simulink model "probnik_1"  (R2019a)
settings: Solver=FixedStepAuto  StartTime=0.0  StopTime=4  FixedStep=1e-5  RelTol=1e-3  EnableMultiTasking=on
values from neighbouring files (symbols this model uses):
  b1 = [3.31578564644 0.905199348927 -1.07588481903 -9.39754581451 6.51989841461 -7.39431810379 -7.98054647446 -7.51470994949 -2.46217346191 -2.60606265068 0.634998142719 -7.34759140015 ... (20 elements, 1x20)]    [b1.mat]
  b2 = [-8.908867836 -6.37810707092 -8.66125679016 -6.19361543655 -8.59416675568 -9.12425804138 -8.47231483459 -9.20506572723 -8.79118919373 -9.36305236816 -9.80707740784 -1.32926535606 ... (15 elements, 1x15)]    [b2.mat]
  b3 = 0.566753208637    [b3.mat]
  w1 = [-3.38608121872 -1.61282348633 -0.811974227428 -26.1486988068 -5.43596601486 -2.50496292114 -2.73406887054 -1.47529745102 -13.9745950699 -4.77835845947 -8.42057037354 -10.048833847 ... (100 elements, 5x20)]    [w1.mat]    (also in w1d.mat = [-28.5484638214 -28.3087368011 -16.2038860321 -18.8476390839)
  w2 = [-1.73702144623 -0.185042783618 -1.43662083149 5.53469181061 0.114013127983 -6.10858488083 1.57797574997 1.2862662077 -7.84612417221 -0.614148855209 -15.9998350143 -5.41085386276 ... (300 elements, 20x15)]    [w2.mat]    (also in w2d.mat = [-15.8134098053 -19.7163829803 -21.1157608032 -0.21424435079)
  w3 = [0.296215087175 2.04968070984 0.382735908031 1.65471422672 0.95603877306]    [w3.mat]    (also in w3d.mat = [-2.66624140739 1.28664553165 0.95645904541 -5.20410871506 2)
libraries: powerlib x33, simulink x14, powerlib_meascontrol x2, neural x2
settings Model: Creator=Андрей  LastModifiedBy=70810
settings DataIOCC: LimitDataPoints=on  SaveFormat=Array  ReturnWorkspaceOutputs=off
settings OptimizationCC: LifeSpan=inf
settings DebuggingCC: SolverPrmCheckMsg=warning  SFUnexpectedBacktrackingDiag=warning  SFNoUnconditionalDefaultTransitionDiag=warning  SFExecutionAtInitializationDiag=none  ArithmeticOperatorsInVariantConditions=warning
settings HardwareCC: ProdBitPerPointer=32  ProdBitPerSizeT=32  ProdBitPerPtrDiffT=32  ProdLargestAtomicFloat=None  ProdIntDivRoundTo=Undefined  ProdEndianess=Unspecified  ProdWordSize=32  ProdHWDeviceType=32-bit Generic
settings ModelReferenceCC: PropagateSignalLabelsOutOfModel=off
settings SFSimCC: SimUseLocalCustomCode=off
settings RTWCC: RTWUseLocalCustomCode=off
settings CodeAppCC: StateflowObjectComments=on
settings GRTTargetCC: TargetLangStandard=C89/C90 (ANSI)  GeneratePreprocessorConditionals=Disable all
settings ConfigComp: CovMetricSettings=dw  CovHtmlReporting=on  CovSaveCumulativeToWorkspaceVar=on  CovSaveSingleToWorkspaceVar=on  CovExternalEMLEnable=off  CovSFcnEnable=off
settings SimscapeCC: SimscapeNormalizeSystem=off

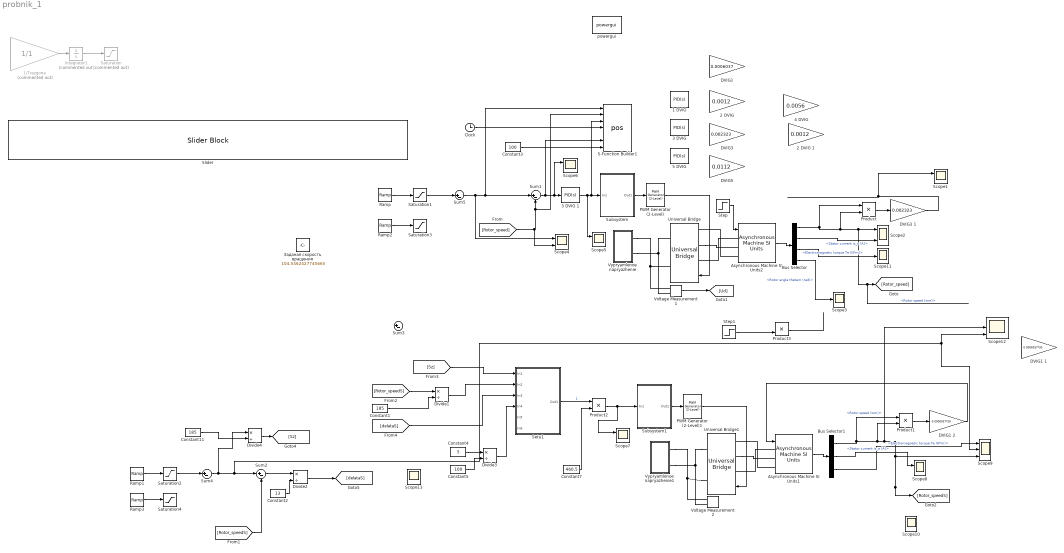
== system probnik_1 ==
  "1 DVIG " : simulink/Continuous/PID Controller  Controller=PID  Form=Parallel  TimeDomain=Continuous-time  SampleTime=-1  IntegratorMethod=Forward Euler  FilterMethod=Forward Euler  ControllerParametersSource=internal  P=1  I=60  D=0.004  UseFilter=on  N=100  TunerSelectOption=Transfer Function Based (PID Tuner App)  InitialConditionSource=internal  InitialConditionForIntegrator=0  InitialConditionForFilter=0  DifferentiatorICPrevScaledInput=0  ExternalReset=none  TrackingMode=off  Kt=1  LimitOutput=off  UpperSaturationLimit=inf  LowerSaturationLimit=-inf  LinearizeAsGain=on  AntiWindupMode=none  Kb=1  POutMin=[]  POutMax=[]  IOutMin=[]  IOutMax=[]  DOutMin=[]  DOutMax=[]  NOutMin=[]  NOutMax=[]  SumOutMin=[]  SumOutMax=[]  SaturationOutMin=[]  SaturationOutMax=[]  PParamMin=[]  PParamMax=[]  IParamMin=[]  IParamMax=[]  DParamMin=[]  DParamMax=[]  NParamMin=[]  NParamMax=[]  KbParamMin=[]  KbParamMax=[]  KtParamMin=[]  KtParamMax=[]  KbOutMin=[]  KbOutMax=[]  KtOutMin=[]  KtOutMax=[]  IntegratorOutMin=[]  IntegratorOutMax=[]  FilterOutMin=[]  FilterOutMax=[]  SumI1OutMin=[]  SumI1OutMax=[]  SumI2OutMin=[]  SumI2OutMax=[]  SumI3OutMin=[]  SumI3OutMax=[]  SumI4OutMin=[]  SumI4OutMax=[]  SumDOutMin=[]  SumDOutMax=[]  DifferentiatorOutMin=[]  DifferentiatorOutMax=[]  FilterDiffOutCoefMin=[]  FilterDiffOutCoefMax=[]  ReciprocalOutMin=[]  ReciprocalOutMax=[]  SumDenOutMin=[]  SumDenOutMax=[]  SumNumOutMin=[]  SumNumOutMax=[]  DivideOutMin=[]  DivideOutMax=[]  IntegratorContinuousStateAttributes=''  IntegratorStateMustResolveToSignalObject=off  IntegratorRTWStateStorageClass=Auto  FilterContinuousStateAttributes=''  FilterStateMustResolveToSignalObject=off  FilterRTWStateStorageClass=Auto  ParallelPVariant=InternalParameters  IdealPVariant=Disabled  IVariant=InternalParameters  DVariant=InternalParameters  IntegratorVariant=Continuous  SatVariant=Disabled  AWVariant=Passthrough  PCopyVariant=Disabled  TRVariant=Disabled  FdbkBlocksVariant=Forward  IdealPFdbkVariant=Disabled  SatFdbkVariant=Disabled  DerivativeFilterVariant=ContFilter  NVariant=InternalParameters  NCopyVariant=Disabled  FilterICVariant=InternalICsFilter  IntegratorICVariant=InternalICs  ExternalResetVariant=Disabled  TRSumVariant=Passthrough  SumFdbkVariant=Disabled  SumVariant=Sum_PID
  1/Trazgona : Gain  Commented=on  Gain=1/1
  "2 DVIG " : Gain  Gain=0.0012
  2 DVIG 1 : Gain  Gain=0.0012
  "3 DVIG " : simulink/Continuous/PID Controller  Controller=PID  Form=Parallel  TimeDomain=Continuous-time  SampleTime=-1  IntegratorMethod=Forward Euler  FilterMethod=Forward Euler  ControllerParametersSource=internal  P=1.8  I=35  D=0  UseFilter=on  N=100  TunerSelectOption=Transfer Function Based (PID Tuner App)  InitialConditionSource=internal  InitialConditionForIntegrator=0  InitialConditionForFilter=0  DifferentiatorICPrevScaledInput=0  ExternalReset=none  TrackingMode=off  Kt=1  LimitOutput=off  UpperSaturationLimit=inf  LowerSaturationLimit=-inf  LinearizeAsGain=on  AntiWindupMode=none  Kb=1  POutMin=[]  POutMax=[]  IOutMin=[]  IOutMax=[]  DOutMin=[]  DOutMax=[]  NOutMin=[]  NOutMax=[]  SumOutMin=[]  SumOutMax=[]  SaturationOutMin=[]  SaturationOutMax=[]  PParamMin=[]  PParamMax=[]  IParamMin=[]  IParamMax=[]  DParamMin=[]  DParamMax=[]  NParamMin=[]  NParamMax=[]  KbParamMin=[]  KbParamMax=[]  KtParamMin=[]  KtParamMax=[]  KbOutMin=[]  KbOutMax=[]  KtOutMin=[]  KtOutMax=[]  IntegratorOutMin=[]  IntegratorOutMax=[]  FilterOutMin=[]  FilterOutMax=[]  SumI1OutMin=[]  SumI1OutMax=[]  SumI2OutMin=[]  SumI2OutMax=[]  SumI3OutMin=[]  SumI3OutMax=[]  SumI4OutMin=[]  SumI4OutMax=[]  SumDOutMin=[]  SumDOutMax=[]  DifferentiatorOutMin=[]  DifferentiatorOutMax=[]  FilterDiffOutCoefMin=[]  FilterDiffOutCoefMax=[]  ReciprocalOutMin=[]  ReciprocalOutMax=[]  SumDenOutMin=[]  SumDenOutMax=[]  SumNumOutMin=[]  SumNumOutMax=[]  DivideOutMin=[]  DivideOutMax=[]  IntegratorContinuousStateAttributes=''  IntegratorStateMustResolveToSignalObject=off  IntegratorRTWStateStorageClass=Auto  FilterContinuousStateAttributes=''  FilterStateMustResolveToSignalObject=off  FilterRTWStateStorageClass=Auto  ParallelPVariant=InternalParameters  IdealPVariant=Disabled  IVariant=InternalParameters  DVariant=InternalParameters  IntegratorVariant=Continuous  SatVariant=Disabled  AWVariant=Passthrough  PCopyVariant=Disabled  TRVariant=Disabled  FdbkBlocksVariant=Forward  IdealPFdbkVariant=Disabled  SatFdbkVariant=Disabled  DerivativeFilterVariant=ContFilter  NVariant=InternalParameters  NCopyVariant=Disabled  FilterICVariant=InternalICsFilter  IntegratorICVariant=InternalICs  ExternalResetVariant=Disabled  TRSumVariant=Passthrough  SumFdbkVariant=Disabled  SumVariant=Sum_PID
  3 DVIG 1 : simulink/Continuous/PID Controller  Controller=PID  Form=Parallel  TimeDomain=Continuous-time  SampleTime=-1  IntegratorMethod=Forward Euler  FilterMethod=Forward Euler  ControllerParametersSource=internal  P=1.8  I=35  D=0  UseFilter=on  N=100  TunerSelectOption=Transfer Function Based (PID Tuner App)  InitialConditionSource=internal  InitialConditionForIntegrator=0  InitialConditionForFilter=0  DifferentiatorICPrevScaledInput=0  ExternalReset=none  TrackingMode=off  Kt=1  LimitOutput=off  UpperSaturationLimit=inf  LowerSaturationLimit=-inf  LinearizeAsGain=on  AntiWindupMode=none  Kb=1  POutMin=[]  POutMax=[]  IOutMin=[]  IOutMax=[]  DOutMin=[]  DOutMax=[]  NOutMin=[]  NOutMax=[]  SumOutMin=[]  SumOutMax=[]  SaturationOutMin=[]  SaturationOutMax=[]  PParamMin=[]  PParamMax=[]  IParamMin=[]  IParamMax=[]  DParamMin=[]  DParamMax=[]  NParamMin=[]  NParamMax=[]  KbParamMin=[]  KbParamMax=[]  KtParamMin=[]  KtParamMax=[]  KbOutMin=[]  KbOutMax=[]  KtOutMin=[]  KtOutMax=[]  IntegratorOutMin=[]  IntegratorOutMax=[]  FilterOutMin=[]  FilterOutMax=[]  SumI1OutMin=[]  SumI1OutMax=[]  SumI2OutMin=[]  SumI2OutMax=[]  SumI3OutMin=[]  SumI3OutMax=[]  SumI4OutMin=[]  SumI4OutMax=[]  SumDOutMin=[]  SumDOutMax=[]  DifferentiatorOutMin=[]  DifferentiatorOutMax=[]  FilterDiffOutCoefMin=[]  FilterDiffOutCoefMax=[]  ReciprocalOutMin=[]  ReciprocalOutMax=[]  SumDenOutMin=[]  SumDenOutMax=[]  SumNumOutMin=[]  SumNumOutMax=[]  DivideOutMin=[]  DivideOutMax=[]  IntegratorContinuousStateAttributes=''  IntegratorStateMustResolveToSignalObject=off  IntegratorRTWStateStorageClass=Auto  FilterContinuousStateAttributes=''  FilterStateMustResolveToSignalObject=off  FilterRTWStateStorageClass=Auto  ParallelPVariant=InternalParameters  IdealPVariant=Disabled  IVariant=InternalParameters  DVariant=InternalParameters  IntegratorVariant=Continuous  SatVariant=Disabled  AWVariant=Passthrough  PCopyVariant=Disabled  TRVariant=Disabled  FdbkBlocksVariant=Forward  IdealPFdbkVariant=Disabled  SatFdbkVariant=Disabled  DerivativeFilterVariant=ContFilter  NVariant=InternalParameters  NCopyVariant=Disabled  FilterICVariant=InternalICsFilter  IntegratorICVariant=InternalICs  ExternalResetVariant=Disabled  TRSumVariant=Passthrough  SumFdbkVariant=Disabled  SumVariant=Sum_PID
  "4 DVIG " : Gain  Gain=0.0056
  "5 DVIG " : simulink/Continuous/PID Controller  Controller=PID  Form=Parallel  TimeDomain=Continuous-time  SampleTime=-1  IntegratorMethod=Forward Euler  FilterMethod=Forward Euler  ControllerParametersSource=internal  P=2.3  I=33  D=0  UseFilter=on  N=100  TunerSelectOption=Transfer Function Based (PID Tuner App)  InitialConditionSource=internal  InitialConditionForIntegrator=0  InitialConditionForFilter=0  DifferentiatorICPrevScaledInput=0  ExternalReset=none  TrackingMode=off  Kt=1  LimitOutput=off  UpperSaturationLimit=inf  LowerSaturationLimit=-inf  LinearizeAsGain=on  AntiWindupMode=none  Kb=1  POutMin=[]  POutMax=[]  IOutMin=[]  IOutMax=[]  DOutMin=[]  DOutMax=[]  NOutMin=[]  NOutMax=[]  SumOutMin=[]  SumOutMax=[]  SaturationOutMin=[]  SaturationOutMax=[]  PParamMin=[]  PParamMax=[]  IParamMin=[]  IParamMax=[]  DParamMin=[]  DParamMax=[]  NParamMin=[]  NParamMax=[]  KbParamMin=[]  KbParamMax=[]  KtParamMin=[]  KtParamMax=[]  KbOutMin=[]  KbOutMax=[]  KtOutMin=[]  KtOutMax=[]  IntegratorOutMin=[]  IntegratorOutMax=[]  FilterOutMin=[]  FilterOutMax=[]  SumI1OutMin=[]  SumI1OutMax=[]  SumI2OutMin=[]  SumI2OutMax=[]  SumI3OutMin=[]  SumI3OutMax=[]  SumI4OutMin=[]  SumI4OutMax=[]  SumDOutMin=[]  SumDOutMax=[]  DifferentiatorOutMin=[]  DifferentiatorOutMax=[]  FilterDiffOutCoefMin=[]  FilterDiffOutCoefMax=[]  ReciprocalOutMin=[]  ReciprocalOutMax=[]  SumDenOutMin=[]  SumDenOutMax=[]  SumNumOutMin=[]  SumNumOutMax=[]  DivideOutMin=[]  DivideOutMax=[]  IntegratorContinuousStateAttributes=''  IntegratorStateMustResolveToSignalObject=off  IntegratorRTWStateStorageClass=Auto  FilterContinuousStateAttributes=''  FilterStateMustResolveToSignalObject=off  FilterRTWStateStorageClass=Auto  ParallelPVariant=InternalParameters  IdealPVariant=Disabled  IVariant=InternalParameters  DVariant=InternalParameters  IntegratorVariant=Continuous  SatVariant=Disabled  AWVariant=Passthrough  PCopyVariant=Disabled  TRVariant=Disabled  FdbkBlocksVariant=Forward  IdealPFdbkVariant=Disabled  SatFdbkVariant=Disabled  DerivativeFilterVariant=ContFilter  NVariant=InternalParameters  NCopyVariant=Disabled  FilterICVariant=InternalICsFilter  IntegratorICVariant=InternalICs  ExternalResetVariant=Disabled  TRSumVariant=Passthrough  SumFdbkVariant=Disabled  SumVariant=Sum_PID
  Asynchronous Machine SI Units1 : powerlib/Machines/Asynchronous Machine SI Units  RotorType=Squirrel-cage  PresetModel="06:  150 HP 460 V 60Hz 1785 RPM"  MechanicalLoad=Torque Tm  ShowDetailedParameters=on  ReferenceFrame=Rotor  Units=SI  MeasurementBus=off  NominalParameters=[1.119e+05 460 60]  Stator=[0.0302 0.000283]  Rotor=[0.01721 0.000283]  Cage1=[ 0.022 0.226/377]  Cage2=[ 0.022 0.226/377]  Lm=0.01095  Mechanical=[2 0.02154 2]  PolePairs=2  InitialConditions=[1 0 0 0 0 0 0 0]  SimulateSaturation=off  Saturation=[14.03593122, 27.81365428, 53.79336849, 72.68890987, 97.98006896, 148.6815601, 215.7428561, 302.9841135, 420.4778367 ; 230, 322, 414, 460, 506, 552, 598, 644, 690]  LoadFlowParameters=1492000  TsPowergui=0  TsBlock=-1  IterativeModel=Trapezoidal non iterative  IterativeDiscreteModel=Trapezoidal non iterative  Pmec=0
      settings: SourceProductName=Simscape Electrical
  Asynchronous Machine SI Units2 : powerlib/Machines/Asynchronous Machine SI Units  RotorType=Squirrel-cage  PresetModel="03:  20 HP  460 V 60Hz 1760 RPM"  MechanicalLoad=Torque Tm  ShowDetailedParameters=on  ReferenceFrame=Rotor  Units=SI  MeasurementBus=off  NominalParameters=[1.492e+04 460 60]  Stator=[0.2761 0.002191]  Rotor=[0.1645 0.002191]  Cage1=[ 0.022 0.226/377]  Cage2=[ 0.022 0.226/377]  Lm=0.07614  Mechanical=[0.1 0.01771 2]  PolePairs=2  InitialConditions=[1 0 0 0 0 0 0 0]  SimulateSaturation=off  Saturation=[14.03593122, 27.81365428, 53.79336849, 72.68890987, 97.98006896, 148.6815601, 215.7428561, 302.9841135, 420.4778367 ; 230, 322, 414, 460, 506, 552, 598, 644, 690]  LoadFlowParameters=1492000  TsPowergui=0  TsBlock=-1  IterativeModel=Trapezoidal non iterative  IterativeDiscreteModel=Trapezoidal non iterative  Pmec=0
      settings: SourceProductName=Simscape Electrical
  Bus Selector : BusSelector  OutputSignals=Mechanical.Rotor speed (wm),Stator measurements.Stator current is_a (A),Mechanical.Electromagnetic torque Te (N*m),Mechanical.Rotor angle thetam (rad)
  Bus Selector1 : BusSelector  OutputSignals=Mechanical.Rotor speed (wm),Stator measurements.Stator current is_a (A),Mechanical.Electromagnetic torque Te (N*m)
  Clock : Clock
  Constant1 : Constant  Value=185
  Constant11 : Constant  Value=185
  Constant2 : Constant  Value=13
  Constant3 : Constant  Value=100
  Constant4 : Constant  Value=5
  Constant5 : Constant  Value=100
  Constant7 : Constant  Value=460.5
  "DVIG1 " : Gain  Gain=0.0006037
  DVIG1 1 : Gain  Gain=0.0006037*30
  DVIG1 2 : Gain  Gain=0.0006037*30
  "DVIG3 " : Gain  Gain=0.002323
  DVIG3 1 : Gain  Gain=0.002323
  "DVIG5 " : Gain  Gain=0.0112
  Divide{1..4} (4 alike) : Product  Inputs=*/
  Integrator1 : Integrator  Commented=on
  PWM Generator (2-Level) : powerlib_meascontrol/Pulse & Signal Generators/PWM Generator (2-Level)  ModulatorType=Three-phase bridge (6 pulses)  ModulatorMode=Unsynchronized  Fc=1500  Pc=90  nF=27  MinMax="[ 0  1000 ]"  SamplingTechnique=Natural  ModulatingSignals=off  m=0.8  Freq=60  Phase=0  Ts=1e-5  ShowCarrierOutport=off
  PWM Generator (2-Level)1 : powerlib_meascontrol/Pulse & Signal Generators/PWM Generator (2-Level)  ModulatorType=Three-phase bridge (6 pulses)  ModulatorMode=Unsynchronized  Fc=1500  Pc=90  nF=27  MinMax="[ 0  1000 ]"  SamplingTechnique=Natural  ModulatingSignals=off  m=0.8  Freq=60  Phase=0  Ts=1e-5  ShowCarrierOutport=off
  Product{,1..3} (4 alike) : Product
  Ramp : simulink/Sources/Ramp  slope=183  start=0.1  InitialOutput=0
  Ramp1 : simulink/Sources/Ramp  slope=183  start=0.1  InitialOutput=0
  Ramp2 : simulink/Sources/Ramp  slope=183  start=1.5  InitialOutput=0
  Ramp3 : simulink/Sources/Ramp  slope=1830  start=1.6  InitialOutput=0
  S-Function Builder1 : S-Function  InitFcn=try, set_param(gcb,'FunctionName','pos'), end  FunctionName=pos  SFunctionModules=pos_wrapper Aray  SFunctionDeploymentMode=off  EnableBusSupport=off  mask(S-Function Builder){}
      mask help: Simulink:masks:SFunctionBuilder_MD
      mask init:
      | val = [[.9  0.75 0.75 1 1 .9 .9 1]',[1 1 0.75 0.75 .9 .9 1 .9]'];try , sys = get_param(gcb,'SfunBuilderFcnName');if isempty(sys), sys = get_param(gcb,'FunctionName'); end,catch, sys = get_param(gcb,'FunctionName'); end
      settings: CopyFcn=set_param(gcbh,'LinkStatus','none')  PreSaveFcn=try, set_param(gcb,'FunctionName','pos'), end  OpenFcn=sfunctionwizard(gcbh)
      mask Display: plot(val(:,1),val(:,2)),disp(sys), port_label('input',1,'u0'), port_label('input',2,'u1'), port_label('input',3,'u2'), port_label('input',4,'u3'), port_label('input',5,'u4'), port_label('input',6,'u5'), port_label('input',7,'u6'), port_label('output',1,'y0')
  Saturation : Saturate  Commented=on  UpperLimit=380  LowerLimit=0
  Saturation{1..4} (4 alike) : Saturate  UpperLimit=183  LowerLimit=0
  Scope{1..2,4..8,13} (8 alike) : Scope  NumInputPorts=2
  Scope10 : Scope
  Scope11 : Scope
  Scope12 : Scope  NumInputPorts=3
  Scope3 : Scope
  Scope9 : Scope  NumInputPorts=3
  Setu1 : Subsystem
  Slider : SliderBlock  ScaleMax=183
  Step : Step  Time=0.8  After=79  SampleTime=0
  Step1 : Step  Time=1.5  Before=1  After=0.1  SampleTime=0
  Subsystem : Subsystem
  Subsystem1 : Subsystem
  Sum{1..5} (5 alike) : Sum  Inputs=|+-
  Universal Bridge : powerlib/Power Electronics/Universal Bridge  Arms=3  SnubberResistance=1e5  SnubberCapacitance=inf  Device=IGBT / Diodes  Ron=1e-3  Lon=0  ForwardVoltages="[  0  0  ]"  ForwardVoltage=0  GTOparameters=[ 10e-6 , 20e-6 ]  IGBTparameters=[ 1e-6 , 2e-6 ]  Measurements=None  Measurements_2=None  converterType=Rectifier
      settings: SourceProductName=Simscape Electrical
  Universal Bridge1 : powerlib/Power Electronics/Universal Bridge  Arms=3  SnubberResistance=1e5  SnubberCapacitance=inf  Device=IGBT / Diodes  Ron=1e-3  Lon=0  ForwardVoltages="[  0  0  ]"  ForwardVoltage=0  GTOparameters=[ 10e-6 , 20e-6 ]  IGBTparameters=[ 1e-6 , 2e-6 ]  Measurements=None  Measurements_2=None  converterType=Rectifier
      settings: SourceProductName=Simscape Electrical
  Voltage Measurement1 : powerlib/Measurements/Voltage Measurement  PhasorSimulation=off  OutputType=Complex  PSBequivalent=0
      settings: SourceProductName=Simscape Electrical
  Voltage Measurement2 : powerlib/Measurements/Voltage Measurement  PhasorSimulation=off  OutputType=Complex  PSBequivalent=0
      settings: SourceProductName=Simscape Electrical
  Vypryamlenoe napryazhenie : Subsystem
  Vypryamlenoe napryazhenie1 : Subsystem
  powergui : powerlib/powergui  Priority=1  SimulationMode=Continuous  SampleTime=2e-5  frequency=60  Iterations=50  frequencyindice=0  Pbase=100e6  ErrMax=1e-4  UnitsV=kV  UnitsW=MW  buscounter=0  FunctionMessages=off  echomessages=off  EnableUseOfTLC=off  CurrentSourceSwitches=on  DisableSnubberDevices=off  DisableRonSwitches=off  DisableVfSwitches=off  DisplayEquations=off  AutomaticDiscreteSolvers=off  SolverType=Tustin  Interpol=off  ExternalGateDelay=off  methode=off  Ts=0  x0status=blocks  SPID=off  SwTol=0  HookPort=off  NonlinearTolerance=1e-4  nMaxIteration=100  ContinueOnMaxIteration=off  RestoreLinks=warning  ResistiveCurrentMeasurement=off  Frange=[0:2:500]  Ylog=off  Xlog=on  ShowGrid=off  save=off  variable=ZData  structure=0  ZoomFFT=off  StartTime=0.0  cycles=1  DisplayStyle=1  fundamental=60  FreqAxis=off  MaxFrequency=1000  frequencyindicesteady=1  RmsSteady=1  display=off
      settings: SourceProductName=Simscape Electrical
  "Заданая скорость вращения " : Constant  Value=104.5462427745665
  wires:
  Asynchronous Machine SI Units2/1 -> Bus Selector/1
  Product/1 -> DVIG3 1/1
  Bus Selector/3 -> Scope11/1  "<Electromagnetic torque Te (N*m)>"
  Bus Selector/1 -> Product/2, [Rotor_speed], Scope2/1, Product/1  "<Rotor speed (wm)>"
  DVIG3 1/1 -> Scope1/1
  Bus Selector/2 -> Scope2/2  "<Stator current is_a (A)>"
  PWM Generator (2-Level)/1 -> Universal Bridge/1
  Sum1/1 -> S-Function Builder1/6, 3 DVIG 1/1, Scope6/1
  [Rotor_speed] -> Scope4/2, S-Function Builder1/2, Sum1/2
  Voltage Measurement1/1 -> [Ud]
  Integrator1/1 -> Saturation/1
  1/Trazgona/1 -> Integrator1/1
  3 DVIG 1/1 -> Scope5/1, S-Function Builder1/3, Subsystem/1(In1)
  Subsystem/1(Out1) -> PWM Generator (2-Level)/1
  Ramp/1 -> Saturation1/1
  Bus Selector/4 -> Scope3/1  "<Rotor angle thetam (rad)>"
  Clock/1 -> S-Function Builder1/4
  PWM Generator (2-Level)1/1 -> Universal Bridge1/1
  Bus Selector1/3 -> Scope9/1  "<Electromagnetic torque Te (N*m)>"
  Subsystem1/1(Out1) -> PWM Generator (2-Level)1/1
  Bus Selector1/2 -> Scope8/1  "<Stator current is_a (A)>"
  Bus Selector1/1 -> Product1/1, Product1/2, Scope12/2, [Rotor_speedS], Scope9/3  "<Rotor speed (wm)>"
  Asynchronous Machine SI Units1/1 -> Bus Selector1/1
  Product1/1 -> DVIG1 2/1
  DVIG1 2/1 -> Asynchronous Machine SI Units1/1
  Setu1/1(Out1) -> Product2/1  "1"
  Constant7/1 -> Product2/2
  Constant11/1 -> Divide4/2
  Divide4/1 -> [Sz]
  Ramp1/1 -> Saturation2/1
  Sum2/1 -> Divide2/1
  [Rotor_speedS] -> Sum2/2
  [Rotor_speedS] -> Divide1/1
  Constant1/1 -> Divide1/2
  Divide1/1 -> Setu1/2(In2)
  [Sz] -> Setu1/1(In1)
  Constant2/1 -> Divide2/2
  Divide2/1 -> [delataS]
  [delataS] -> Setu1/3(In3)
  Product2/1 -> Scope7/1, Subsystem1/1(In1)
  Saturation2/1 -> Sum4/1
  Sum4/1 -> Divide4/1, Scope9/2, Scope12/3, Sum2/1
  Saturation1/1 -> Sum5/1
  Sum5/1 -> Scope4/1, S-Function Builder1/1, Sum1/1
  Constant3/1 -> S-Function Builder1/7
  Constant4/1 -> Divide3/1
  Constant5/1 -> Divide3/2
  Divide3/1 -> Setu1/4(In4)
  Ramp2/1 -> Saturation3/1
  Ramp3/1 -> Saturation4/1
  Step/1 -> Asynchronous Machine SI Units2/1
  Step1/1 -> Product3/2
  Product3/1 -> ?
  connections:
  Asynchronous Machine SI Units2/LConn1 -- Universal Bridge/LConn1
  Asynchronous Machine SI Units2/LConn3 -- Universal Bridge/LConn3
  Universal Bridge/LConn2 -- Asynchronous Machine SI Units2/LConn2
  Vypryamlenoe napryazhenie/RConn2 -- Voltage Measurement1/LConn2 -- Universal Bridge/RConn2
  Voltage Measurement1/LConn1 -- Vypryamlenoe napryazhenie/RConn1 -- Universal Bridge/RConn1
  Universal Bridge1/RConn1 -- Voltage Measurement2/LConn1 -- Vypryamlenoe napryazhenie1/RConn1
  Universal Bridge1/RConn2 -- Vypryamlenoe napryazhenie1/RConn2 -- Voltage Measurement2/LConn2
  Asynchronous Machine SI Units1/LConn1 -- Universal Bridge1/LConn1
  Universal Bridge1/LConn2 -- Asynchronous Machine SI Units1/LConn2
  Asynchronous Machine SI Units1/LConn3 -- Universal Bridge1/LConn3

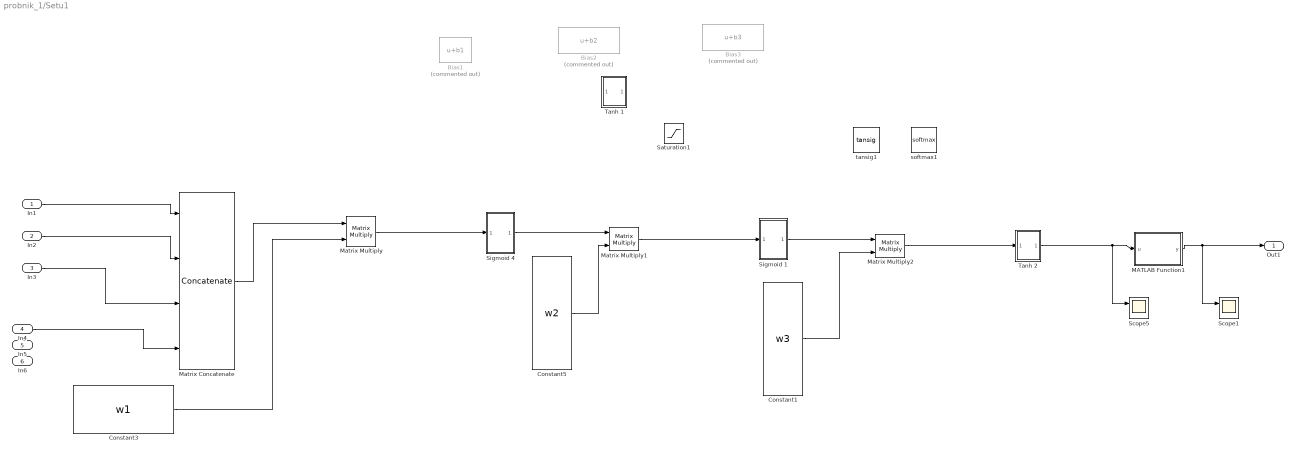
== system probnik_1/Setu1 ==
  In1 : Inport
  In2 : Inport  Port=2
  In3 : Inport  Port=3
  In4 : Inport  Port=4
  In5 : Inport  Port=5
  In6 : Inport  Port=6
  Bias1 : Bias  Commented=on  Bias=b1
  Bias2 : Bias  Commented=on  Bias=b2
  Bias3 : Bias  Commented=on  Bias=b3
  Constant1 : Constant  Value=w3  VectorParams1D=off
  Constant3 : Constant  Value=w1  VectorParams1D=off
  Constant5 : Constant  Value=w2  VectorParams1D=off
  MATLAB Function1 : MATLAB Function  TreatAsAtomicUnit=on
  Matrix Concatenate : Concatenate  NumInputs=4  Mode=Multidimensional array  ConcatenateDimension=2
  Matrix Multiply : Product  Multiplication=Matrix(*)
  Matrix Multiply1 : Product  Multiplication=Matrix(*)
  Matrix Multiply2 : Product  Multiplication=Matrix(*)
  Saturation1 : Saturate  UpperLimit=inf  LowerLimit=0
  Scope1 : Scope  NumInputPorts=2
  Scope5 : Scope  NumInputPorts=2
  Sigmoid 1 : Subsystem
  Sigmoid 4 : Subsystem
  Tanh 1 : Subsystem
  Tanh 2 : Subsystem
  softmax1 : neural/Transfer Functions/softmax
      settings: SourceProductName=MATLAB Runtime - Deep Learning Toolbox  SourceProductBaseCode=Missing
  tansig1 : neural/Transfer Functions/tansig
      settings: SourceProductName=MATLAB Runtime - Deep Learning Toolbox  SourceProductBaseCode=Missing
  Out1 : Outport
  wires:
  Sigmoid 4/1(Out1) -> Matrix Multiply1/1
  Sigmoid 1/1(Out1) -> Matrix Multiply2/1
  Constant1/1 -> Matrix Multiply2/2
  Constant3/1 -> Matrix Multiply/2
  Constant5/1 -> Matrix Multiply1/2
  In1/1 -> Matrix Concatenate/1
  Matrix Concatenate/1 -> Matrix Multiply/1
  In2/1 -> Matrix Concatenate/2
  In3/1 -> Matrix Concatenate/3
  In4/1 -> Matrix Concatenate/4
  Matrix Multiply/1 -> Sigmoid 4/1(In1)
  Matrix Multiply1/1 -> Sigmoid 1/1(In1)
  Matrix Multiply2/1 -> Tanh 2/1(In1)
  Tanh 2/1(Out1) -> MATLAB Function1/1(u), Scope5/1
  MATLAB Function1/1(y) -> Scope1/1, Out1/1

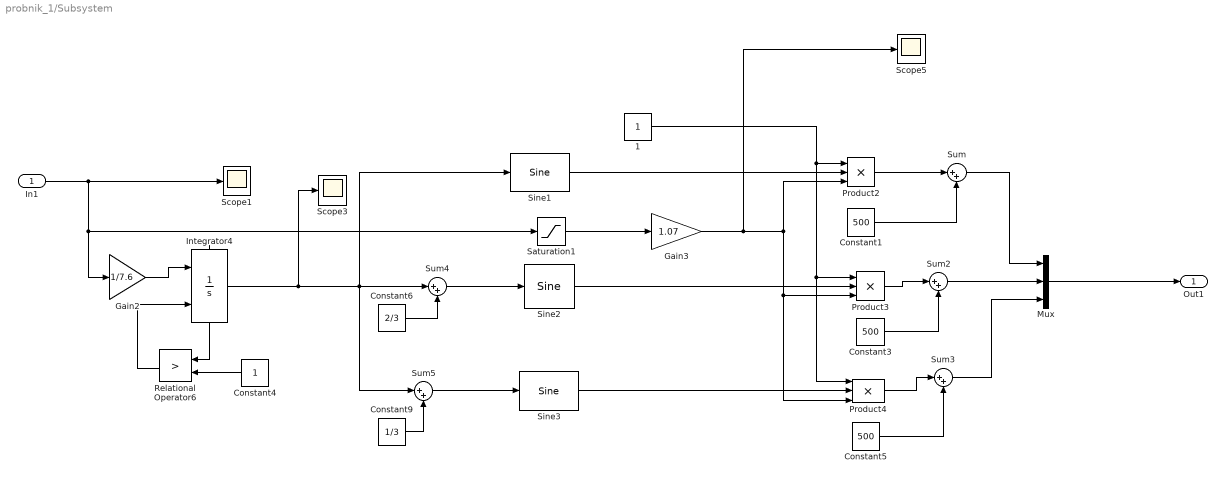
== system probnik_1/Subsystem ==
  In1 : Inport
  " 1" : Constant
  Constant1 : Constant  Value=500
  Constant3 : Constant  Value=500
  Constant4 : Constant
  Constant5 : Constant  Value=500
  Constant6 : Constant  Value=2/3
  Constant9 : Constant  Value=1/3
  Gain2 : Gain  Gain=1/7.6
  Gain3 : Gain  Gain=1.07
  Integrator4 : Integrator  ExternalReset=rising  ShowStatePort=on
  Mux : Mux  Inputs=3
  Product2 : Product  Inputs=3
  Product3 : Product  Inputs=3
  Product4 : Product  Inputs=3
  Relational Operator6 : RelationalOperator  Operator=>  RndMeth=Nearest  InputSameDT=on
  Saturation1 : Saturate  UpperLimit=650  LowerLimit=-650
  Scope1 : Scope
  Scope3 : Scope
  Scope5 : Scope
  Sine1 : simulink/Lookup Tables/Sine  Formula=sin(2*pi*u)  NumDataPoints=(2^5)+1  OutputWordLength=16  InternalRulePriority=Speed
      settings: SourceProductName=Simulink
  Sine2 : simulink/Lookup Tables/Sine  Formula=sin(2*pi*u)  NumDataPoints=(2^5)+1  OutputWordLength=16  InternalRulePriority=Speed
      settings: SourceProductName=Simulink
  Sine3 : simulink/Lookup Tables/Sine  Formula=sin(2*pi*u)  NumDataPoints=(2^5)+1  OutputWordLength=16  InternalRulePriority=Speed
      settings: SourceProductName=Simulink
  Sum{,2..5} (5 alike) : Sum  Inputs=|++
  Out1 : Outport
  wires:
  In1/1 -> Saturation1/1, Gain2/1, Scope1/1
  Integrator4/State -> Relational Operator6/1
  Gain3/1 -> Scope5/1, Product2/3, Product4/3, Product3/3
  Relational Operator6/1 -> Integrator4/2
  Product3/1 -> Sum2/1
  Constant5/1 -> Sum3/2
  Sine1/1 -> Product2/2
  Sine2/1 -> Product3/2
  Product4/1 -> Sum3/1
  Constant6/1 -> Sum4/2
  Constant1/1 -> Sum/2
  Constant9/1 -> Sum5/2
  Sum4/1 -> Sine2/1
  Sum5/1 -> Sine3/1
  Gain2/1 -> Integrator4/1
  Sum3/1 -> Mux/3
  Sum/1 -> Mux/1
  Constant4/1 -> Relational Operator6/2
  Constant3/1 -> Sum2/2
  Sine3/1 -> Product4/2
  Integrator4/1 -> Scope3/1, Sine1/1, Sum5/1, Sum4/1
  Saturation1/1 -> Gain3/1
  Sum2/1 -> Mux/2
  Product2/1 -> Sum/1
  " 1"/1 -> Product4/1, Product3/1, Product2/1
  Mux/1 -> Out1/1

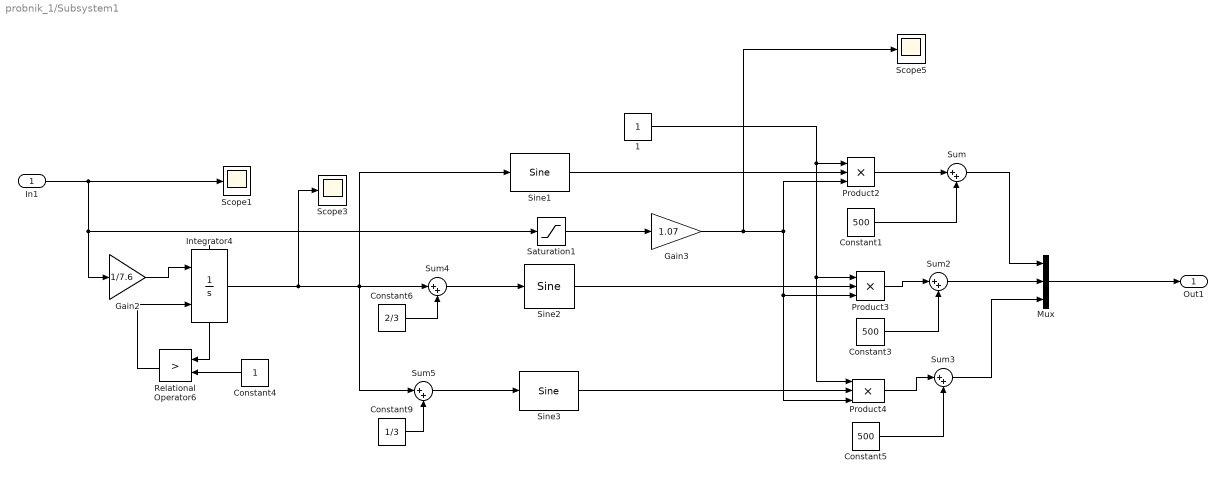
== system probnik_1/Subsystem1 ==
  In1 : Inport
  " 1" : Constant
  Constant1 : Constant  Value=500
  Constant3 : Constant  Value=500
  Constant4 : Constant
  Constant5 : Constant  Value=500
  Constant6 : Constant  Value=2/3
  Constant9 : Constant  Value=1/3
  Gain2 : Gain  Gain=1/7.6
  Gain3 : Gain  Gain=1.07
  Integrator4 : Integrator  ExternalReset=rising  ShowStatePort=on
  Mux : Mux  Inputs=3
  Product2 : Product  Inputs=3
  Product3 : Product  Inputs=3
  Product4 : Product  Inputs=3
  Relational Operator6 : RelationalOperator  Operator=>  RndMeth=Nearest  InputSameDT=on
  Saturation1 : Saturate  UpperLimit=650  LowerLimit=-650
  Scope1 : Scope
  Scope3 : Scope
  Scope5 : Scope
  Sine1 : simulink/Lookup Tables/Sine  Formula=sin(2*pi*u)  NumDataPoints=(2^5)+1  OutputWordLength=16  InternalRulePriority=Speed
      settings: SourceProductName=Simulink
  Sine2 : simulink/Lookup Tables/Sine  Formula=sin(2*pi*u)  NumDataPoints=(2^5)+1  OutputWordLength=16  InternalRulePriority=Speed
      settings: SourceProductName=Simulink
  Sine3 : simulink/Lookup Tables/Sine  Formula=sin(2*pi*u)  NumDataPoints=(2^5)+1  OutputWordLength=16  InternalRulePriority=Speed
      settings: SourceProductName=Simulink
  Sum{,2..5} (5 alike) : Sum  Inputs=|++
  Out1 : Outport
  wires:
  In1/1 -> Saturation1/1, Gain2/1, Scope1/1
  Integrator4/State -> Relational Operator6/1
  Gain3/1 -> Scope5/1, Product2/3, Product4/3, Product3/3
  Relational Operator6/1 -> Integrator4/2
  Product3/1 -> Sum2/1
  Constant5/1 -> Sum3/2
  Sine1/1 -> Product2/2
  Sine2/1 -> Product3/2
  Product4/1 -> Sum3/1
  Constant6/1 -> Sum4/2
  Constant1/1 -> Sum/2
  Constant9/1 -> Sum5/2
  Sum4/1 -> Sine2/1
  Sum5/1 -> Sine3/1
  Gain2/1 -> Integrator4/1
  Sum3/1 -> Mux/3
  Sum/1 -> Mux/1
  Constant4/1 -> Relational Operator6/2
  Constant3/1 -> Sum2/2
  Sine3/1 -> Product4/2
  Integrator4/1 -> Scope3/1, Sine1/1, Sum5/1, Sum4/1
  Saturation1/1 -> Gain3/1
  Sum2/1 -> Mux/2
  Product2/1 -> Sum/1
  " 1"/1 -> Product4/1, Product3/1, Product2/1
  Mux/1 -> Out1/1

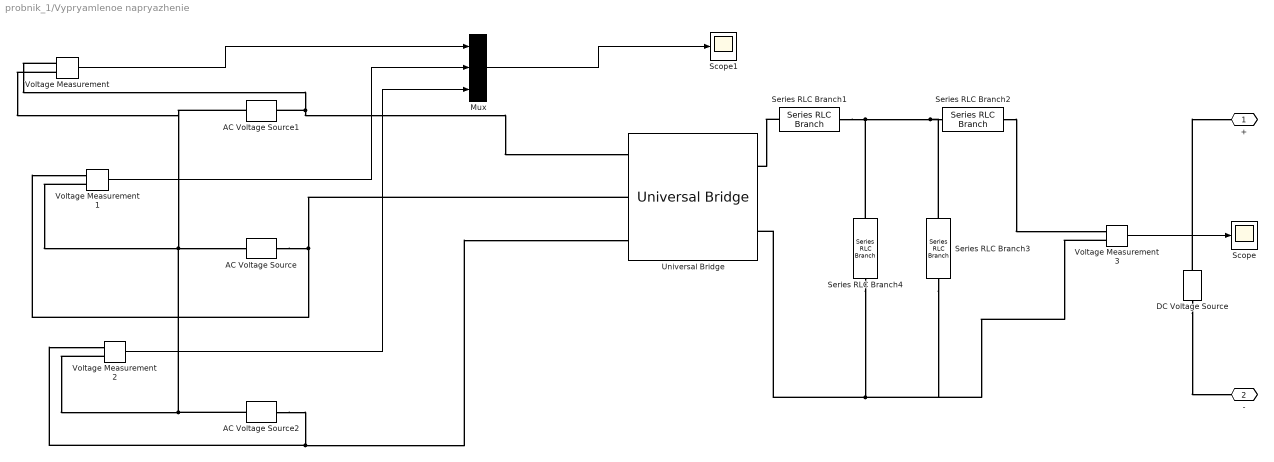
== system probnik_1/Vypryamlenoe napryazhenie ==
  AC Voltage Source : powerlib/Electrical Sources/AC Voltage Source  Amplitude=460  Phase=120  Frequency=120  SampleTime=0  Measurements=None  BusType=swing  Pref=10e3  Qref=0  Qmin=-inf  Qmax=+inf
      settings: SourceProductName=Simscape Electrical
  AC Voltage Source1 : powerlib/Electrical Sources/AC Voltage Source  Amplitude=460  Phase=0  Frequency=120  SampleTime=0  Measurements=None  BusType=swing  Pref=10e3  Qref=0  Qmin=-inf  Qmax=+inf
      settings: SourceProductName=Simscape Electrical
  AC Voltage Source2 : powerlib/Electrical Sources/AC Voltage Source  Amplitude=460  Phase=240  Frequency=120  SampleTime=0  Measurements=None  BusType=swing  Pref=10e3  Qref=0  Qmin=-inf  Qmax=+inf
      settings: SourceProductName=Simscape Electrical
  DC Voltage Source : powerlib/Electrical Sources/DC Voltage Source  Amplitude=900  Measurements=None
      settings: SourceProductName=Simscape Electrical
  Mux : Mux  Inputs=3
  Scope : Scope
  Scope1 : Scope
  Series RLC Branch1 : powerlib/Elements/Series RLC Branch  LConnTagsString=__new0  RConnTagsString=__new0  BranchType=R  Resistance=0.01  Inductance=1e-3  SetiL0=off  InitialCurrent=0  Capacitance=1e-3  Setx0=off  InitialVoltage=0  Measurements=None
      settings: SourceProductName=Simscape Electrical
  Series RLC Branch2 : powerlib/Elements/Series RLC Branch  LConnTagsString=__new0  RConnTagsString=__new0  BranchType=R  Resistance=0.01  Inductance=1e-3  SetiL0=off  InitialCurrent=0  Capacitance=1e-3  Setx0=off  InitialVoltage=0  Measurements=None
      settings: SourceProductName=Simscape Electrical
  Series RLC Branch3 : powerlib/Elements/Series RLC Branch  LConnTagsString=__new0  RConnTagsString=__new0  BranchType=C  Resistance=100  Inductance=1e-3  SetiL0=off  InitialCurrent=0  Capacitance=3e-3  Setx0=off  InitialVoltage=0  Measurements=None
      settings: SourceProductName=Simscape Electrical
  Series RLC Branch4 : powerlib/Elements/Series RLC Branch  LConnTagsString=__new0  RConnTagsString=__new0  BranchType=R  Resistance=1  Inductance=1e-3  SetiL0=off  InitialCurrent=0  Capacitance=1e-3  Setx0=off  InitialVoltage=0  Measurements=None
      settings: SourceProductName=Simscape Electrical
  Universal Bridge : powerlib/Power Electronics/Universal Bridge  Arms=3  SnubberResistance=1e5  SnubberCapacitance=inf  Device=Diodes  Ron=1e-3  Lon=0  ForwardVoltages="[  0  0  ]"  ForwardVoltage=0  GTOparameters=[ 10e-6 , 20e-6 ]  IGBTparameters=[ 1e-6 , 2e-6 ]  Measurements=None  Measurements_2=None  converterType=Rectifier
      settings: SourceProductName=Simscape Electrical
  Voltage Measurement{,1..3} (4 alike) : powerlib/Measurements/Voltage Measurement  PhasorSimulation=off  OutputType=Complex  PSBequivalent=0
      settings: SourceProductName=Simscape Electrical
  + : PMIOPort  Side=Right
  - : PMIOPort  Port=2  Side=Right
  wires:
  Voltage Measurement/1 -> Mux/1
  Voltage Measurement2/1 -> Mux/3
  Mux/1 -> Scope1/1
  Voltage Measurement1/1 -> Mux/2
  Voltage Measurement3/1 -> Scope/1
  connections:
  AC Voltage Source2/LConn1 -- Voltage Measurement/LConn2 -- AC Voltage Source1/LConn1 -- AC Voltage Source/LConn1 -- Voltage Measurement1/LConn2 -- Voltage Measurement2/LConn2
  AC Voltage Source2/RConn1 -- Universal Bridge/LConn3 -- Voltage Measurement2/LConn1
  Voltage Measurement3/LConn2 -- Series RLC Branch3/LConn1 -- Series RLC Branch4/LConn1 -- Universal Bridge/RConn2
  AC Voltage Source/RConn1 -- Voltage Measurement1/LConn1 -- Universal Bridge/LConn2
  Series RLC Branch1/LConn1 -- Series RLC Branch4/RConn1 -- Series RLC Branch3/RConn1 -- Series RLC Branch2/RConn1
  Series RLC Branch2/LConn1 -- Voltage Measurement3/LConn1
  Voltage Measurement/LConn1 -- Universal Bridge/LConn1 -- AC Voltage Source1/RConn1
  Series RLC Branch1/RConn1 -- Universal Bridge/RConn1
  DC Voltage Source/RConn1 -- +/RConn1
  DC Voltage Source/LConn1 -- -/RConn1

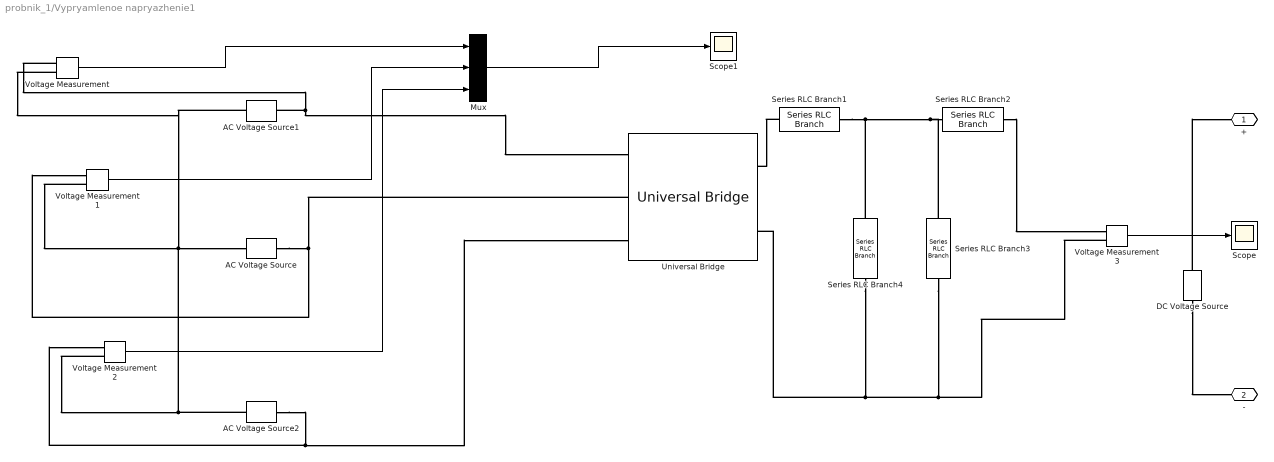
== system probnik_1/Vypryamlenoe napryazhenie1 ==
  AC Voltage Source : powerlib/Electrical Sources/AC Voltage Source  Amplitude=460  Phase=120  Frequency=120  SampleTime=0  Measurements=None  BusType=swing  Pref=10e3  Qref=0  Qmin=-inf  Qmax=+inf
      settings: SourceProductName=Simscape Electrical
  AC Voltage Source1 : powerlib/Electrical Sources/AC Voltage Source  Amplitude=460  Phase=0  Frequency=120  SampleTime=0  Measurements=None  BusType=swing  Pref=10e3  Qref=0  Qmin=-inf  Qmax=+inf
      settings: SourceProductName=Simscape Electrical
  AC Voltage Source2 : powerlib/Electrical Sources/AC Voltage Source  Amplitude=460  Phase=240  Frequency=120  SampleTime=0  Measurements=None  BusType=swing  Pref=10e3  Qref=0  Qmin=-inf  Qmax=+inf
      settings: SourceProductName=Simscape Electrical
  DC Voltage Source : powerlib/Electrical Sources/DC Voltage Source  Amplitude=900  Measurements=None
      settings: SourceProductName=Simscape Electrical
  Mux : Mux  Inputs=3
  Scope : Scope
  Scope1 : Scope
  Series RLC Branch1 : powerlib/Elements/Series RLC Branch  LConnTagsString=__new0  RConnTagsString=__new0  BranchType=R  Resistance=0.01  Inductance=1e-3  SetiL0=off  InitialCurrent=0  Capacitance=1e-3  Setx0=off  InitialVoltage=0  Measurements=None
      settings: SourceProductName=Simscape Electrical
  Series RLC Branch2 : powerlib/Elements/Series RLC Branch  LConnTagsString=__new0  RConnTagsString=__new0  BranchType=R  Resistance=0.01  Inductance=1e-3  SetiL0=off  InitialCurrent=0  Capacitance=1e-3  Setx0=off  InitialVoltage=0  Measurements=None
      settings: SourceProductName=Simscape Electrical
  Series RLC Branch3 : powerlib/Elements/Series RLC Branch  LConnTagsString=__new0  RConnTagsString=__new0  BranchType=C  Resistance=100  Inductance=1e-3  SetiL0=off  InitialCurrent=0  Capacitance=3e-3  Setx0=off  InitialVoltage=0  Measurements=None
      settings: SourceProductName=Simscape Electrical
  Series RLC Branch4 : powerlib/Elements/Series RLC Branch  LConnTagsString=__new0  RConnTagsString=__new0  BranchType=R  Resistance=1  Inductance=1e-3  SetiL0=off  InitialCurrent=0  Capacitance=1e-3  Setx0=off  InitialVoltage=0  Measurements=None
      settings: SourceProductName=Simscape Electrical
  Universal Bridge : powerlib/Power Electronics/Universal Bridge  Arms=3  SnubberResistance=1e5  SnubberCapacitance=inf  Device=Diodes  Ron=1e-3  Lon=0  ForwardVoltages="[  0  0  ]"  ForwardVoltage=0  GTOparameters=[ 10e-6 , 20e-6 ]  IGBTparameters=[ 1e-6 , 2e-6 ]  Measurements=None  Measurements_2=None  converterType=Rectifier
      settings: SourceProductName=Simscape Electrical
  Voltage Measurement{,1..3} (4 alike) : powerlib/Measurements/Voltage Measurement  PhasorSimulation=off  OutputType=Complex  PSBequivalent=0
      settings: SourceProductName=Simscape Electrical
  + : PMIOPort  Side=Right
  - : PMIOPort  Port=2  Side=Right
  wires:
  Voltage Measurement/1 -> Mux/1
  Voltage Measurement2/1 -> Mux/3
  Mux/1 -> Scope1/1
  Voltage Measurement1/1 -> Mux/2
  Voltage Measurement3/1 -> Scope/1
  connections:
  AC Voltage Source2/LConn1 -- Voltage Measurement/LConn2 -- AC Voltage Source1/LConn1 -- AC Voltage Source/LConn1 -- Voltage Measurement1/LConn2 -- Voltage Measurement2/LConn2
  AC Voltage Source2/RConn1 -- Universal Bridge/LConn3 -- Voltage Measurement2/LConn1
  Voltage Measurement3/LConn2 -- Series RLC Branch3/LConn1 -- Series RLC Branch4/LConn1 -- Universal Bridge/RConn2
  AC Voltage Source/RConn1 -- Voltage Measurement1/LConn1 -- Universal Bridge/LConn2
  Series RLC Branch1/LConn1 -- Series RLC Branch4/RConn1 -- Series RLC Branch3/RConn1 -- Series RLC Branch2/RConn1
  Series RLC Branch2/LConn1 -- Voltage Measurement3/LConn1
  Voltage Measurement/LConn1 -- Universal Bridge/LConn1 -- AC Voltage Source1/RConn1
  Series RLC Branch1/RConn1 -- Universal Bridge/RConn1
  DC Voltage Source/RConn1 -- +/RConn1
  DC Voltage Source/LConn1 -- -/RConn1

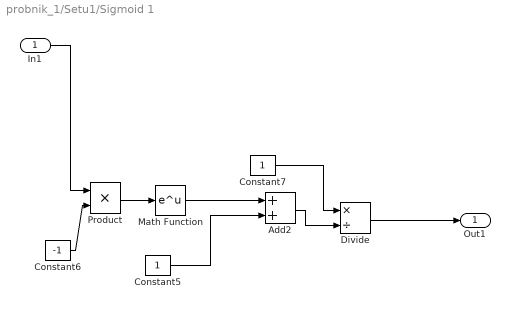
== system probnik_1/Setu1/Sigmoid 1 ==
  In1 : Inport
  Add2 : Sum
  Constant5 : Constant  VectorParams1D=off
  Constant6 : Constant  Value=-1  VectorParams1D=off
  Constant7 : Constant  VectorParams1D=off
  Divide : Product  Inputs=*/
  Math Function : Math  SaturateOnIntegerOverflow=on
  Product : Product
  Out1 : Outport
  wires:
  Product/1 -> Math Function/1
  Math Function/1 -> Add2/1
  Constant5/1 -> Add2/2
  Constant7/1 -> Divide/1
  Constant6/1 -> Product/2
  In1/1 -> Product/1
  Add2/1 -> Divide/2
  Divide/1 -> Out1/1

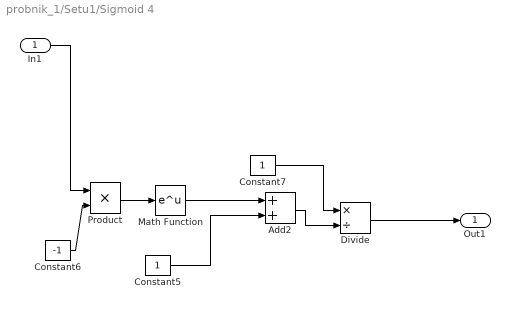
== system probnik_1/Setu1/Sigmoid 4 ==
  In1 : Inport
  Add2 : Sum
  Constant5 : Constant  VectorParams1D=off
  Constant6 : Constant  Value=-1  VectorParams1D=off
  Constant7 : Constant  VectorParams1D=off
  Divide : Product  Inputs=*/
  Math Function : Math  SaturateOnIntegerOverflow=on
  Product : Product
  Out1 : Outport
  wires:
  Product/1 -> Math Function/1
  Math Function/1 -> Add2/1
  Constant5/1 -> Add2/2
  Constant7/1 -> Divide/1
  Constant6/1 -> Product/2
  In1/1 -> Product/1
  Add2/1 -> Divide/2
  Divide/1 -> Out1/1

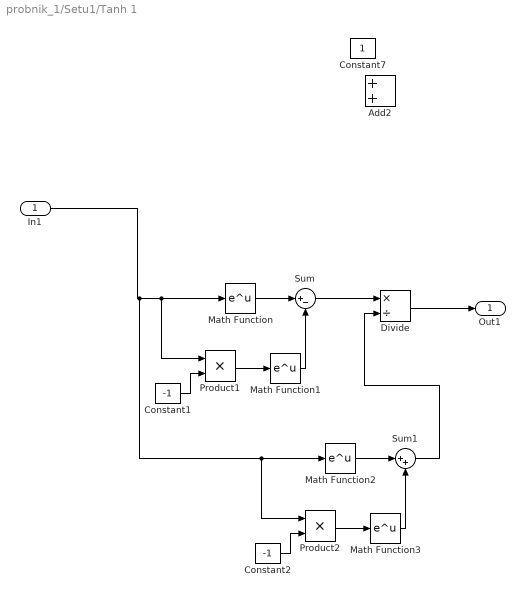
== system probnik_1/Setu1/Tanh 1 ==
  In1 : Inport
  Add2 : Sum
  Constant1 : Constant  Value=-1  VectorParams1D=off
  Constant2 : Constant  Value=-1  VectorParams1D=off
  Constant7 : Constant  VectorParams1D=off
  Divide : Product  Inputs=*/
  Math Function{,1..3} (4 alike) : Math  SaturateOnIntegerOverflow=on
  Product1 : Product
  Product2 : Product
  Sum : Sum  Inputs=|+-
  Sum1 : Sum  Inputs=|++
  Out1 : Outport
  wires:
  Divide/1 -> Out1/1
  Sum1/1 -> Divide/2
  Product2/1 -> Math Function3/1
  Math Function2/1 -> Sum1/1
  In1/1 -> Math Function/1, Product1/1, Math Function2/1, Product2/1
  Constant2/1 -> Product2/2
  Math Function3/1 -> Sum1/2
  Sum/1 -> Divide/1
  Math Function1/1 -> Sum/2
  Constant1/1 -> Product1/2
  Math Function/1 -> Sum/1
  Product1/1 -> Math Function1/1
  ? -> Add2/2

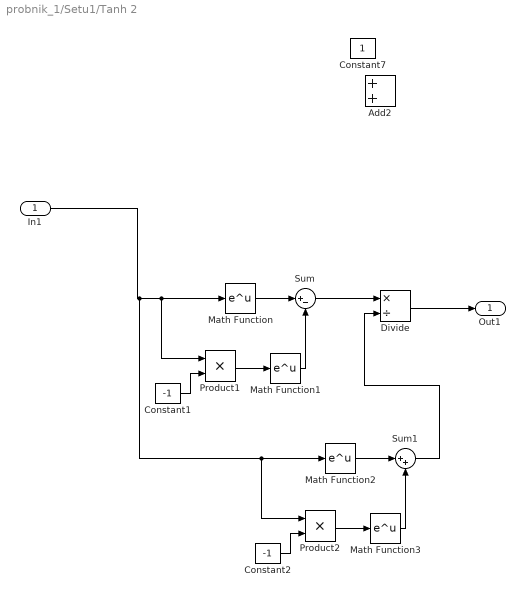
== system probnik_1/Setu1/Tanh 2 ==
  In1 : Inport
  Add2 : Sum
  Constant1 : Constant  Value=-1  VectorParams1D=off
  Constant2 : Constant  Value=-1  VectorParams1D=off
  Constant7 : Constant  VectorParams1D=off
  Divide : Product  Inputs=*/
  Math Function{,1..3} (4 alike) : Math  SaturateOnIntegerOverflow=on
  Product1 : Product
  Product2 : Product
  Sum : Sum  Inputs=|+-
  Sum1 : Sum  Inputs=|++
  Out1 : Outport
  wires:
  ? -> Add2/2
  Product1/1 -> Math Function1/1
  Math Function/1 -> Sum/1
  Constant1/1 -> Product1/2
  Math Function1/1 -> Sum/2
  Sum/1 -> Divide/1
  Math Function3/1 -> Sum1/2
  Constant2/1 -> Product2/2
  In1/1 -> Product2/1, Math Function2/1, Product1/1, Math Function/1
  Math Function2/1 -> Sum1/1
  Product2/1 -> Math Function3/1
  Sum1/1 -> Divide/2
  Divide/1 -> Out1/1

== matlab function probnik_1/Setu1/MATLAB Function1 ==
  data: u input; y output

function y = fcn(u)
if(u<0.01)
u=0;
end
y = u;
